simulink model "Simulation"  (Simulink 6.0)
settings: Solver=ode3  StartTime=0.0  StopTime=100  FixedStep=1e-2  RelTol=1e-3
undefined symbols (not defined in the file or in its folder): sigbuilder_block
libraries: simulink x3
CloseFcn:
  | rtwprivate ssgencode ModelCloseRequest Simulation
settings Model: LastModifiedBy=Yann
settings OptimizationCC: InlineInvariantSignals=off

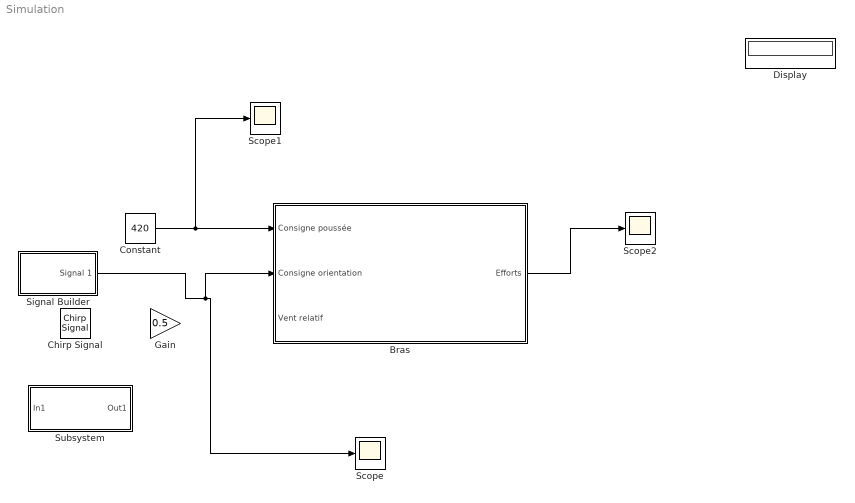
== system Simulation ==
  Bras : Subsystem
  Chirp Signal : simulink/Sources/Chirp Signal  f1=0.1  T=100  f2=0.1
  Constant : Constant  Value=420
  Display : Display
  Gain : Gain  Gain=0.5
  Scope : Scope
  Scope1 : Scope
  Scope2 : Scope
      settings: SaveName=ScopeData2
  Signal Builder : Subsystem  Tag=STV Subsys  LoadFcn=sigbuilder_block('load');  StartFcn=sigbuilder_block('start');  StopFcn=sigbuilder_block('stop');  ClipboardFcn=sigbuilder_block('clipboard');  mask(Sigbuilder block){}
      mask help: Sigbuilder GUI
      mask init:
      | if ~strcmp(get_param(bdroot(gcbh),'SimulationStatus'),'stopped') tuvar = sigbuilder_block('maskInit'); end
      settings: CopyFcn=sigbuilder_block('copy');  DeleteFcn=sigbuilder_block('delete');  ModelCloseFcn=sigbuilder_block('modelClose');  PreSaveFcn=sigbuilder_block('preSave');  NameChangeFcn=sigbuilder_block('namechange');  OpenFcn=sigbuilder_block('open',[50.2759 50.2759 854.069 399.724 ]);  CloseFcn=sigbuilder_block('close');
      mask Display: plot(0,0,100,100,[10,10,40,40,10],[80,20,20,80,80],[40,10],[50,50], [40,27,10],[65,72,56],[40,25,25,10],[28,28,43,43]);
  Subsystem : Subsystem
  wires:
  Constant/1 -> Bras/1(Consigne poussée), Scope1/1
  Bras/1(Efforts) -> Scope2/1
  Signal Builder/1(Signal 1) -> Scope/1, Bras/2(Consigne orientation)

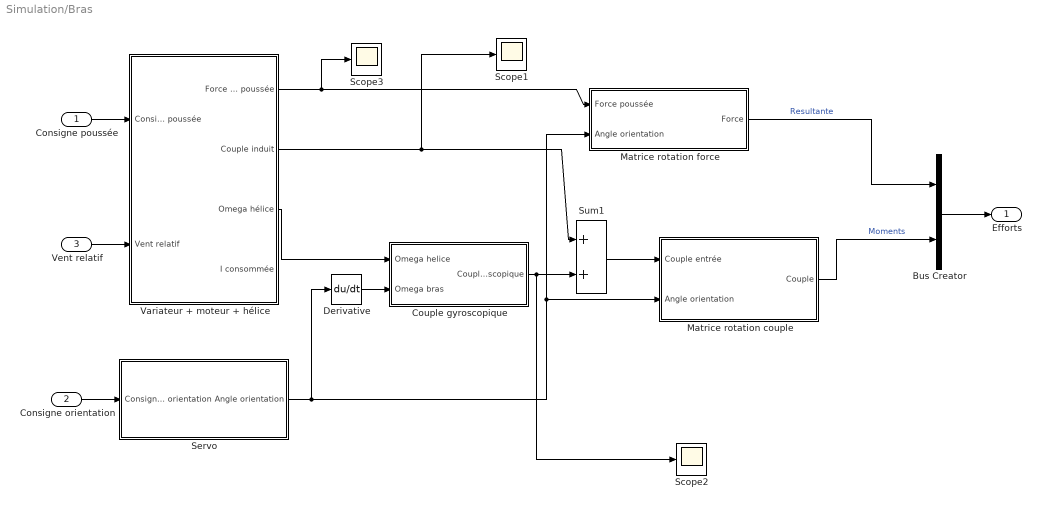
== system Simulation/Bras ==
  Consigne poussée : Inport  Port=1  LatchInput=off
  Consigne orientation : Inport  Port=2  LatchInput=off
  Vent relatif : Inport  Port=3  LatchInput=off
  Bus Creator : BusCreator  DialogController=Simulink.DDGSource_Bus  Inputs=2
  Couple gyroscopique : Subsystem
  Derivative : Derivative
  Matrice rotation couple : Subsystem
  Matrice rotation force : Subsystem
  Scope1 : Scope
      settings: SaveName=ScopeData4
  Scope2 : Scope
      settings: SaveName=ScopeData5
  Scope3 : Scope
      settings: SaveName=ScopeData3
  Servo : Subsystem
  Sum1 : Sum
  Variateur + moteur + hélice : Subsystem
  Efforts : Outport
  wires:
  Consigne poussée/1 -> Variateur + moteur + hélice/1(Consigne poussée)
  Servo/1(Angle orientation) -> Matrice rotation force/2(Angle orientation), Matrice rotation couple/2(Angle orientation), Derivative/1
  Matrice rotation force/1(Force) -> Bus Creator/1  "Resultante"
  Matrice rotation couple/1(Couple) -> Bus Creator/2  "Moments"
  Variateur + moteur + hélice/1(Force de poussée) -> Matrice rotation force/1(Force poussée), Scope3/1
  Derivative/1 -> Couple gyroscopique/2(Omega bras)
  Variateur + moteur + hélice/3(Omega hélice) -> Couple gyroscopique/1(Omega helice)
  Sum1/1 -> Matrice rotation couple/1(Couple entrée)
  Couple gyroscopique/1(Couple gyroscopique) -> Sum1/2, Scope2/1
  Variateur + moteur + hélice/2(Couple induit) -> Sum1/1, Scope1/1
  Bus Creator/1 -> Efforts/1
  Consigne orientation/1 -> Servo/1(Consigne orientation)
  Vent relatif/1 -> Variateur + moteur + hélice/2(Vent relatif)

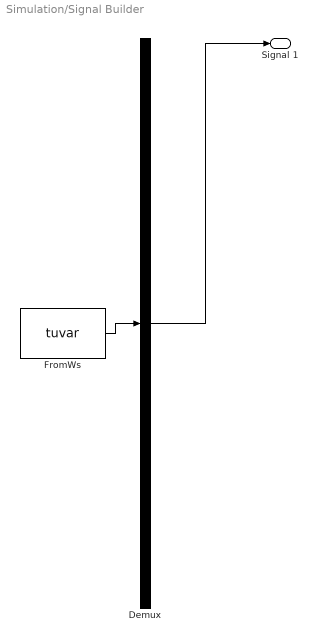
== system Simulation/Signal Builder ==
  Demux : Demux  Tag=STV Demux  Outputs=1
  FromWs : FromWorkspace  Tag=STV FromWs  VariableName=tuvar  SampleTime=0  SigBuilderData=DataTag0  VnvData=DataTag1
      SigBuilderData=|
      | channels.label = 'Signal 1'
      | channels.allXData = {[0 20 87.7 100]}
      | channels.allYData = {[0 0.395 0.395 0]}
      | dataSet.timeRange = [0 100]
      | dataSet.name = 'Group 1'
  Signal 1 : Outport  Tag=STV Outport
  wires:
  Demux/1 -> Signal 1/1
  FromWs/1 -> Demux/1

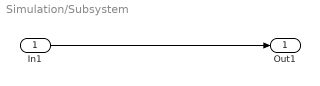
== system Simulation/Subsystem ==
  In1 : Inport  Port=1  LatchInput=off
  Out1 : Outport
  wires:
  In1/1 -> Out1/1

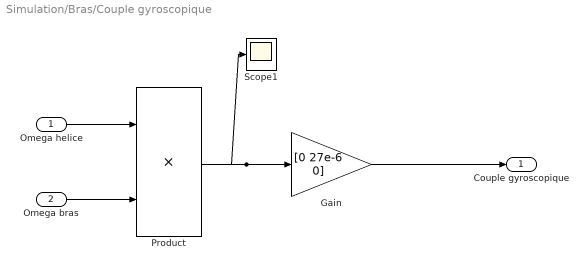
== system Simulation/Bras/Couple gyroscopique ==
  Omega helice : Inport  Port=1  LatchInput=off
  Omega bras : Inport  Port=2  LatchInput=off
  Gain : Gain  Gain=[0 27e-6 0]
  Product : Product  RndMeth=Zero
  Scope1 : Scope
      settings: SaveName=ScopeData6
  Couple gyroscopique : Outport
  wires:
  Omega helice/1 -> Product/1
  Omega bras/1 -> Product/2
  Product/1 -> Gain/1, Scope1/1
  Gain/1 -> Couple gyroscopique/1

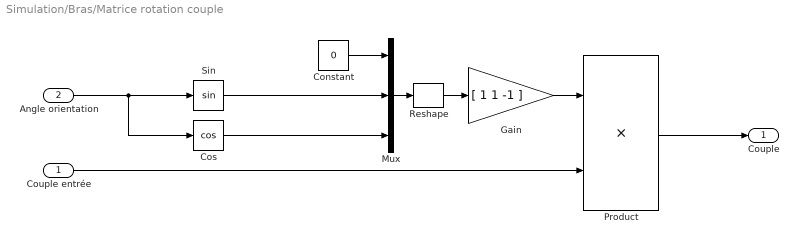
== system Simulation/Bras/Matrice rotation couple ==
  Couple entrée : Inport  Port=1  LatchInput=off
  Angle orientation : Inport  Port=2  LatchInput=off
  Constant : Constant  Value=0
  Cos : Trigonometry  Operator=cos
  Gain : Gain  Gain=[ 1 1 -1 ]
  Mux : Mux  Inputs=3
  Product : Product  RndMeth=Zero
  Reshape : simulink/Math Operations/Reshape  OutputDimensionality=1-D array  OutputDimensions=[1,1]
  Sin : Trigonometry
  Couple : Outport
  wires:
  Angle orientation/1 -> Cos/1, Sin/1
  Constant/1 -> Mux/1
  Cos/1 -> Mux/3
  Sin/1 -> Mux/2
  Mux/1 -> Reshape/1
  Gain/1 -> Product/1
  Couple entrée/1 -> Product/2
  Product/1 -> Couple/1
  Reshape/1 -> Gain/1

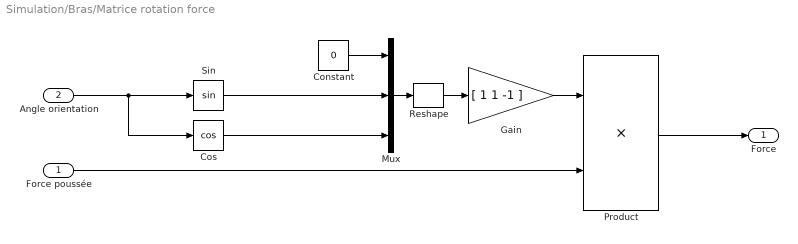
== system Simulation/Bras/Matrice rotation force ==
  Force poussée : Inport  Port=1  LatchInput=off
  Angle orientation : Inport  Port=2  LatchInput=off
  Constant : Constant  Value=0
  Cos : Trigonometry  Operator=cos
  Gain : Gain  Gain=[ 1 1 -1 ]
  Mux : Mux  Inputs=3
  Product : Product  RndMeth=Zero
  Reshape : simulink/Math Operations/Reshape  OutputDimensionality=1-D array  OutputDimensions=[1,1]
  Sin : Trigonometry
  Force : Outport
  wires:
  Angle orientation/1 -> Cos/1, Sin/1
  Constant/1 -> Mux/1
  Cos/1 -> Mux/3
  Sin/1 -> Mux/2
  Mux/1 -> Reshape/1
  Gain/1 -> Product/1
  Force poussée/1 -> Product/2
  Product/1 -> Force/1
  Reshape/1 -> Gain/1

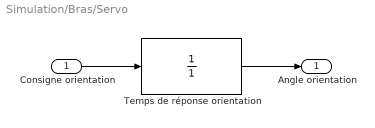
== system Simulation/Bras/Servo ==
  Consigne orientation : Inport  Port=1  LatchInput=off
  Temps de réponse orientation : TransferFcn  Denominator=[ 0 1]
  Angle orientation : Outport
  wires:
  Consigne orientation/1 -> Temps de réponse orientation/1
  Temps de réponse orientation/1 -> Angle orientation/1

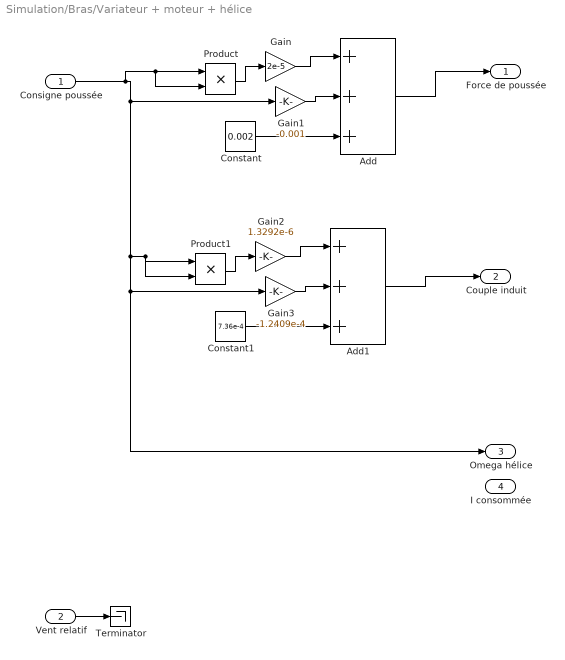
== system Simulation/Bras/Variateur + moteur + hélice ==
  Consigne poussée : Inport  Port=1  LatchInput=off
  Vent relatif : Inport  Port=2  LatchInput=off
  Add : Sum  Inputs=+++  OutScaling=2^-10
  Add1 : Sum  Inputs=+++  OutScaling=2^-10
  Constant : Constant  Value=0.002
  Constant1 : Constant  Value=7.36e-4
  Gain : Gain  Gain=2e-5
  Gain1 : Gain  Gain=-0.001
  Gain2 : Gain  Gain=1.3292e-6
  Gain3 : Gain  Gain=-1.2409e-4
  Product : Product  RndMeth=Zero
  Product1 : Product  RndMeth=Zero
  Terminator : Terminator
  Force de poussée : Outport
  Couple induit : Outport  Port=2
  Omega hélice : Outport  Port=3
  I consommée : Outport  Port=4
  wires:
  Vent relatif/1 -> Terminator/1
  Consigne poussée/1 -> Product/1, Product/2, Gain1/1, Omega hélice/1, Gain3/1, Product1/2, Product1/1
  Product/1 -> Gain/1
  Gain/1 -> Add/1
  Gain1/1 -> Add/2
  Constant/1 -> Add/3
  Add/1 -> Force de poussée/1
  Product1/1 -> Gain2/1
  Gain2/1 -> Add1/1
  Gain3/1 -> Add1/2
  Constant1/1 -> Add1/3
  Add1/1 -> Couple induit/1
